simulink model "NL_Corner_FIw"  (R2016b)
settings: Solver=FixedStepAuto  StartTime=0.0  StopTime=5  FixedStep=0.001  RelTol=1e-3
values from neighbouring files (symbols this model uses):
  AccelError = eye(3)    [SimulinkInit.m]
  C_psi = 3.1176e-5    (= 3.1176e-05)    [ParameterInit.m]
  control_system = CS_LQR    (= 1)    [SimulinkInit.m]
  dPhiMat = [cos(phi_30)/cos(phi_20), -sin(phi_30)/cos(phi_20), 0 ... (first row only)    [ParameterInit.m]
  g = 9.81    [ParameterInit.m]
  GyroError = eye(3)    [SimulinkInit.m]
  I_K_inv = inv(I_K)    [ParameterInit.m]
  I_KO = I_GHO + m_R*(eye(3)*dot(r_1,r_1)-r_1*r_1')                 + m_R*(eye(3)*dot(r_2,r_2)-r_2*r_2')                 + m_R*(eye(3)*dot(r_3,r_3)-r_3*r_3')    [ParameterInit.m]
  I_R1M1 = [3.358e-4, 0, 0; 0, 1.961e-4, 0; 0, 0, 1.681e-4]    [ParameterInit.m]
  I_R2M2 = [1.691e-4, 0, 0; 0, 3.358e-4, 0; 0, 0, 1.961e-4]    [ParameterInit.m]
  I_R3M3 = [1.961e-4, 0, 0; 0, 1.691e-4, 0; 0, 0, 3.358e-4]    [ParameterInit.m]
  I_R_inv = inv(I_R)    [ParameterInit.m]
  Kd = K_unlimited    [LinearSimulationScript.m]    (also in controller_design_lqr.m = KKd * [eye(7), zeros(7,2)]/T_K)
  l_C = 0.066    [ParameterInit.m]
  m = 1.532    [ParameterInit.m]
  phi0 = x0(1:3) + [0; phi_20; phi_30]    [SimulinkInit.m]
  phi_20 = -2*atan(sqrt(2)-sqrt(3))    [ParameterInit.m]
  phi_30 = -pi/4    (= -0.785398163397)    [ParameterInit.m]
  saturation_select = SATURATION_OFF    [LinearSimulationScript.m]    (also in SimulinkInit.m = 2)
  Ta = 0.02    [ParameterInit.m]
  u_K0 = x0(4:6)    [SimulinkInit.m]
  u_R0 = x0(7:9)    [SimulinkInit.m]
  x0 = [0; 0.11; 0.08; 0; 1; -2; 3; -16; 0]    [LinearSimulationScript.m]    (also in SimulinkInit.m = [0; 0.05; 0.02; 0; 0; 0; 0; 0; 0])
  x_offset = [0; 0.02; 0.0; 0; 0; 0; 0; 0; 0]    [SimulinkInit.m]
libraries: vrlib x4, simulink x1
settings Model: Creator=michael  LastModifiedBy=ich

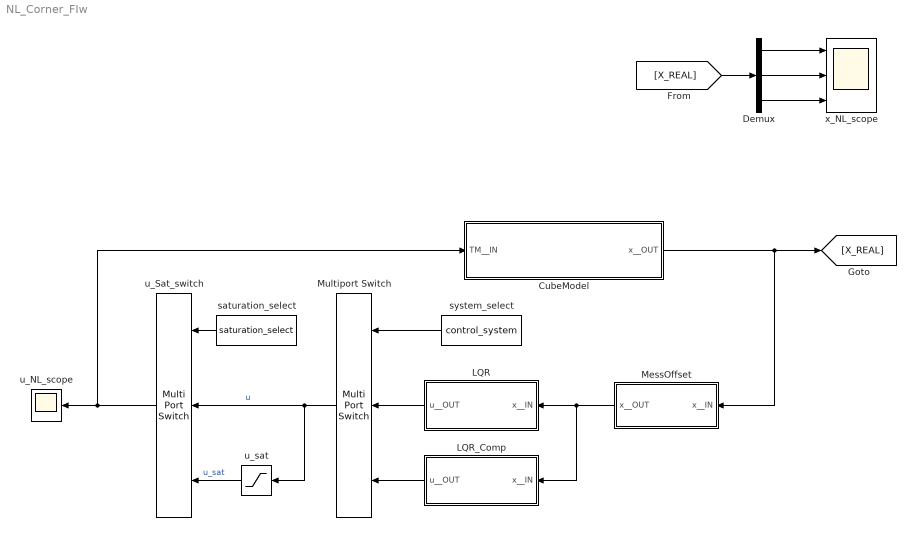
== system NL_Corner_FIw ==
  CubeModel : Subsystem
  Demux : Demux  Outputs=3
  LQR : Subsystem
  LQR_Comp : Subsystem
  MessOffset : Subsystem
  Multiport Switch : MultiPortSwitch  Inputs=2
  saturation_select : Constant  Value=saturation_select
  system_select : Constant  Value=control_system
  u_NL_scope : Scope
  u_Sat_switch : MultiPortSwitch  Inputs=2
  u_sat : Saturate  UpperLimit=0.1  LowerLimit=-0.1
  x_NL_scope : Scope  NumInputPorts=3
  wires:
  MessOffset/1(x__OUT) -> LQR/1(x__IN), LQR_Comp/1(x__IN)
  CubeModel/1(x__OUT) -> [X_REAL], MessOffset/1(x__IN)
  [X_REAL] -> Demux/1
  Demux/1 -> x_NL_scope/1
  Demux/2 -> x_NL_scope/2
  Demux/3 -> x_NL_scope/3
  LQR/1(u__OUT) -> Multiport Switch/2
  LQR_Comp/1(u__OUT) -> Multiport Switch/3
  system_select/1 -> Multiport Switch/1
  u_sat/1 -> u_Sat_switch/3  "u_sat"
  Multiport Switch/1 -> u_Sat_switch/2, u_sat/1  "u"
  saturation_select/1 -> u_Sat_switch/1
  u_Sat_switch/1 -> CubeModel/1(TM__IN), u_NL_scope/1

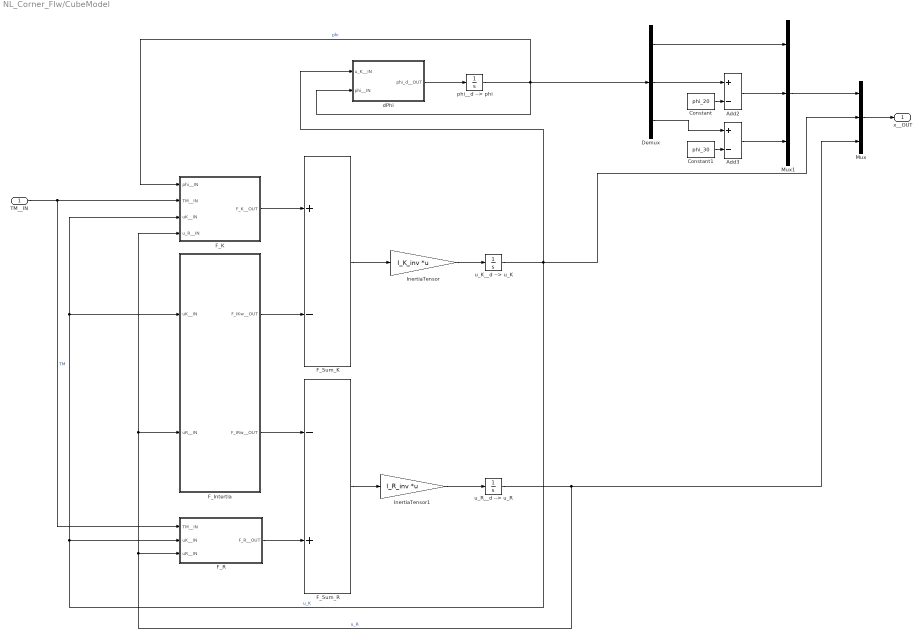
== system NL_Corner_FIw/CubeModel ==
  TM__IN : Inport
  Add2 : Sum  Inputs=+-
  Add3 : Sum  Inputs=+-
  Constant : Constant  Value=phi_20
  Constant1 : Constant  Value=phi_30
  Demux : Demux  Outputs=3
  F_Intertia : Subsystem
  F_K : Subsystem
  F_R : Subsystem
  F_Sum_K : Sum  Inputs=+-
  F_Sum_R : Sum  Inputs=-+
  InertiaTensor : Gain  Gain=I_K_inv  Multiplication=Matrix(K*u) (u vector)
  InertiaTensor1 : Gain  Gain=I_R_inv  Multiplication=Matrix(K*u) (u vector)
  Mux : Mux  Inputs=3
  Mux1 : Mux  Inputs=3
  dPhi : Subsystem
  phi__d --> phi : Integrator  InitialCondition=phi0
  u_K__d --> u_K : Integrator  InitialCondition=u_K0
  u_R__d --> u_R : Integrator  InitialCondition=u_R0
  x__OUT : Outport
  wires:
  u_K__d --> u_K/1 -> F_R/2(uK__IN), F_Intertia/1(uK__IN), F_K/3(uK__IN), dPhi/1(u_K__IN), Mux/2  "u_K"
  u_R__d --> u_R/1 -> F_R/3(uR__IN), F_Intertia/2(uR__IN), F_K/4(u_R__IN), Mux/3  "u_R"
  dPhi/1(phi_d__OUT) -> phi__d --> phi/1
  Mux/1 -> x__OUT/1
  phi__d --> phi/1 -> dPhi/2(phi__IN), F_K/1(phi__IN), Demux/1  "phi"
  Demux/2 -> Add2/1
  Demux/3 -> Add3/1
  Constant1/1 -> Add3/2
  Constant/1 -> Add2/2
  Demux/1 -> Mux1/1
  Add2/1 -> Mux1/2
  Add3/1 -> Mux1/3
  Mux1/1 -> Mux/1
  F_K/1(F_K__OUT) -> F_Sum_K/1
  F_Sum_K/1 -> InertiaTensor/1
  F_R/1(F_R__OUT) -> F_Sum_R/2
  F_Sum_R/1 -> InertiaTensor1/1
  InertiaTensor/1 -> u_K__d --> u_K/1
  InertiaTensor1/1 -> u_R__d --> u_R/1
  TM__IN/1 -> F_K/2(TM__IN), F_R/1(TM__IN)  "TM"
  F_Intertia/2(F_IRw__OUT) -> F_Sum_R/1
  F_Intertia/1(F_IKw__OUT) -> F_Sum_K/2

== system NL_Corner_FIw/LQR ==
  x__IN : Inport  SampleTime=Ta
  Gain : Gain  Gain=-Kd  Multiplication=Matrix(K*u) (u vector)
  u__OUT : Outport
  wires:
  x__IN/1 -> Gain/1
  Gain/1 -> u__OUT/1

== system NL_Corner_FIw/LQR_Comp ==
  x__IN : Inport  SampleTime=Ta
  CompFilter : Subsystem
  Gain : Gain  Gain=-Kd  Multiplication=Matrix(K*u) (u vector)
  u__OUT : Outport
  wires:
  x__IN/1 -> CompFilter/1(x__IN)
  Gain/1 -> u__OUT/1
  CompFilter/1(x__OUT) -> Gain/1

== system NL_Corner_FIw/MessOffset ==
  x__IN : Inport
  Add : Sum  Inputs=+++
  Band-Limited White Noise : simulink/Sources/Band-Limited White Noise  Cov=x_noise  Ts=0.1  seed=[1;2;3;4;5;6;7;8;9]
  Constant : Constant  Value=x_offset
  SensorTilt : Subsystem
  x__OUT : Outport
  wires:
  x__IN/1 -> SensorTilt/1(x__IN)
  Add/1 -> x__OUT/1
  Constant/1 -> Add/2
  Band-Limited White Noise/1 -> Add/3
  SensorTilt/1(x__OUT) -> Add/1

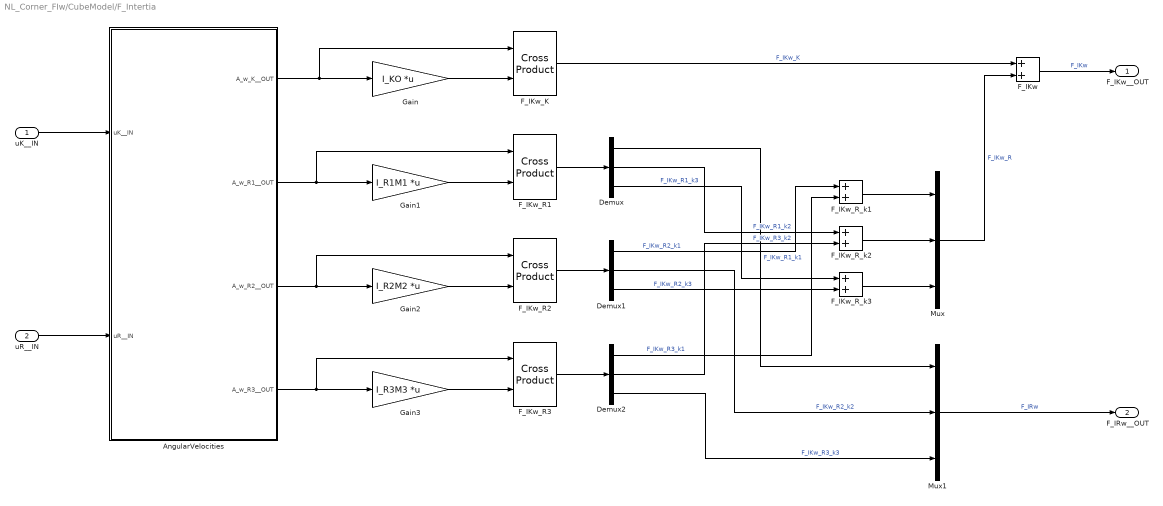
== system NL_Corner_FIw/CubeModel/F_Intertia ==
  uK__IN : Inport
  uR__IN : Inport  Port=2
  AngularVelocities : Subsystem
  Demux : Demux  Outputs=3
  Demux1 : Demux  Outputs=3
  Demux2 : Demux  Outputs=3
  F_IKw : Sum
  F_IKw_K : vrlib/Utilities/Cross Product
  F_IKw_R1 : vrlib/Utilities/Cross Product
  F_IKw_R2 : vrlib/Utilities/Cross Product
  F_IKw_R3 : vrlib/Utilities/Cross Product
  F_IKw_R_k1 : Sum
  F_IKw_R_k2 : Sum
  F_IKw_R_k3 : Sum
  Gain : Gain  Gain=I_KO  Multiplication=Matrix(K*u) (u vector)
  Gain1 : Gain  Gain=I_R1M1  Multiplication=Matrix(K*u) (u vector)
  Gain2 : Gain  Gain=I_R2M2  Multiplication=Matrix(K*u) (u vector)
  Gain3 : Gain  Gain=I_R3M3  Multiplication=Matrix(K*u) (u vector)
  Mux : Mux  Inputs=3
  Mux1 : Mux  Inputs=3
  F_IKw__OUT : Outport
  F_IRw__OUT : Outport  Port=2
  wires:
  uK__IN/1 -> AngularVelocities/1(uK__IN)
  uR__IN/1 -> AngularVelocities/2(uR__IN)
  AngularVelocities/1(A_w_K__OUT) -> F_IKw_K/1, Gain/1
  Gain/1 -> F_IKw_K/2
  AngularVelocities/2(A_w_R1__OUT) -> F_IKw_R1/1, Gain1/1
  Gain1/1 -> F_IKw_R1/2
  AngularVelocities/3(A_w_R2__OUT) -> Gain2/1, F_IKw_R2/1
  Gain2/1 -> F_IKw_R2/2
  AngularVelocities/4(A_w_R3__OUT) -> F_IKw_R3/1, Gain3/1
  Gain3/1 -> F_IKw_R3/2
  F_IKw_R1/1 -> Demux/1
  Demux/1 -> Mux1/1  "F_IKw_R1_k1"
  Demux/2 -> F_IKw_R_k2/1  "F_IKw_R1_k2"
  Demux/3 -> F_IKw_R_k3/1  "F_IKw_R1_k3"
  F_IKw_R2/1 -> Demux1/1
  Demux1/1 -> F_IKw_R_k1/1  "F_IKw_R2_k1"
  Demux1/2 -> Mux1/2  "F_IKw_R2_k2"
  Demux1/3 -> F_IKw_R_k3/2  "F_IKw_R2_k3"
  F_IKw_R3/1 -> Demux2/1
  Demux2/1 -> F_IKw_R_k1/2  "F_IKw_R3_k1"
  Demux2/2 -> F_IKw_R_k2/2  "F_IKw_R3_k2"
  Demux2/3 -> Mux1/3  "F_IKw_R3_k3"
  F_IKw_R_k1/1 -> Mux/1
  F_IKw_R_k3/1 -> Mux/3
  F_IKw_R_k2/1 -> Mux/2
  Mux/1 -> F_IKw/2  "F_IKw_R"
  F_IKw_K/1 -> F_IKw/1  "F_IKw_K"
  F_IKw/1 -> F_IKw__OUT/1  "F_IKw"
  Mux1/1 -> F_IRw__OUT/1  "F_IRw"

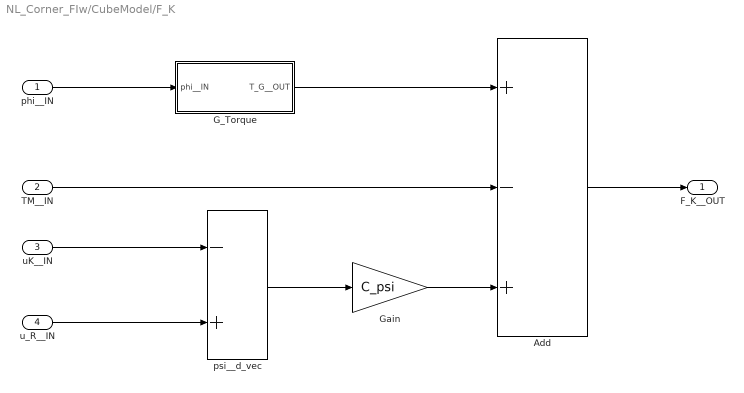
== system NL_Corner_FIw/CubeModel/F_K ==
  phi__IN : Inport
  TM__IN : Inport  Port=2
  uK__IN : Inport  Port=3
  u_R__IN : Inport  Port=4
  Add : Sum  Inputs=+-+
  G_Torque : Subsystem
  Gain : Gain  Gain=C_psi
  psi__d_vec : Sum  Inputs=-+
  F_K__OUT : Outport
  wires:
  phi__IN/1 -> G_Torque/1(phi__IN)
  uK__IN/1 -> psi__d_vec/1
  u_R__IN/1 -> psi__d_vec/2
  psi__d_vec/1 -> Gain/1
  G_Torque/1(T_G__OUT) -> Add/1
  Gain/1 -> Add/3
  TM__IN/1 -> Add/2
  Add/1 -> F_K__OUT/1

== system NL_Corner_FIw/CubeModel/F_R ==
  TM__IN : Inport
  uK__IN : Inport  Port=2
  uR__IN : Inport  Port=3
  Gain : Gain  Gain=C_psi
  TorqueSum : Sum  Inputs=+-
  psi__d_vec : Sum  Inputs=-+
  F_R__OUT : Outport
  wires:
  uR__IN/1 -> psi__d_vec/2
  uK__IN/1 -> psi__d_vec/1
  psi__d_vec/1 -> Gain/1
  TM__IN/1 -> TorqueSum/1
  Gain/1 -> TorqueSum/2
  TorqueSum/1 -> F_R__OUT/1  "F_R"

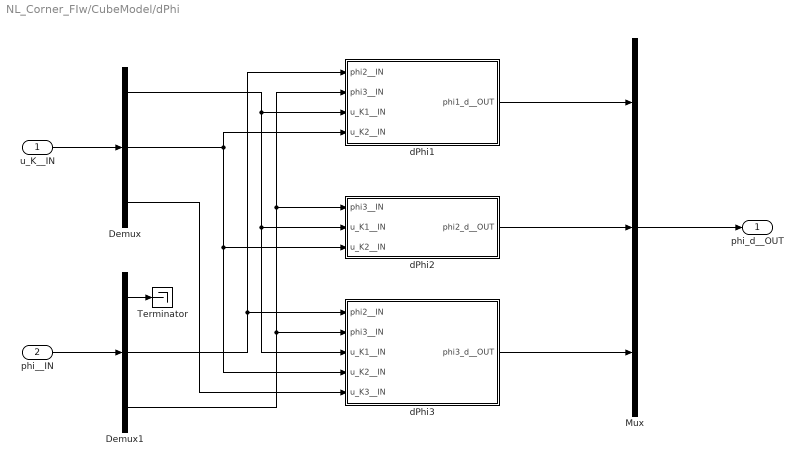
== system NL_Corner_FIw/CubeModel/dPhi ==
  u_K__IN : Inport
  phi__IN : Inport  Port=2
  Demux : Demux  Outputs=3
  Demux1 : Demux  Outputs=3
  Mux : Mux  Inputs=3
  Terminator : Terminator
  dPhi1 : Subsystem
  dPhi2 : Subsystem
  dPhi3 : Subsystem
  phi_d__OUT : Outport
  wires:
  u_K__IN/1 -> Demux/1
  Mux/1 -> phi_d__OUT/1
  phi__IN/1 -> Demux1/1
  dPhi1/1(phi1_d__OUT) -> Mux/1
  dPhi2/1(phi2_d__OUT) -> Mux/2
  dPhi3/1(phi3_d__OUT) -> Mux/3
  Demux1/2 -> dPhi3/1(phi2__IN), dPhi1/1(phi2__IN)
  Demux1/3 -> dPhi3/2(phi3__IN), dPhi2/1(phi3__IN), dPhi1/2(phi3__IN)
  Demux1/1 -> Terminator/1
  Demux/2 -> dPhi2/3(u_K2__IN), dPhi3/4(u_K2__IN), dPhi1/4(u_K2__IN)
  Demux/3 -> dPhi3/5(u_K3__IN)
  Demux/1 -> dPhi1/3(u_K1__IN), dPhi2/2(u_K1__IN), dPhi3/3(u_K1__IN)

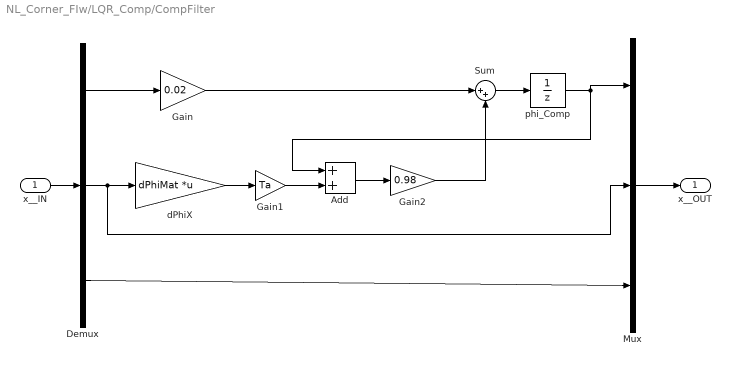
== system NL_Corner_FIw/LQR_Comp/CompFilter ==
  x__IN : Inport
  Add : Sum
  Demux : Demux  Outputs=3
  Gain : Gain  Gain=0.02
  Gain1 : Gain  Gain=Ta
  Gain2 : Gain  Gain=0.98
  Mux : Mux  Inputs=3
  Sum : Sum  Inputs=|++
  dPhiX : Gain  Gain=dPhiMat  Multiplication=Matrix(K*u) (u vector)
  phi_Comp : UnitDelay  InitialCondition=x0(1:3)  SampleTime=0.02
  x__OUT : Outport
  wires:
  x__IN/1 -> Demux/1
  Demux/1 -> Gain/1
  Demux/2 -> Mux/2, dPhiX/1
  dPhiX/1 -> Gain1/1
  Gain1/1 -> Add/2
  Add/1 -> Gain2/1
  Gain/1 -> Sum/1
  Gain2/1 -> Sum/2
  Sum/1 -> phi_Comp/1
  phi_Comp/1 -> Add/1, Mux/1
  Mux/1 -> x__OUT/1
  Demux/3 -> Mux/3

== system NL_Corner_FIw/MessOffset/SensorTilt ==
  x__IN : Inport
  Demux : Demux  Outputs=3
  Gain : Gain  Gain=GyroError  Multiplication=Matrix(K*u) (u vector)
  Gain1 : Gain  Gain=AccelError  Multiplication=Matrix(K*u) (u vector)
  Mux : Mux  Inputs=3
  x__OUT : Outport
  wires:
  x__IN/1 -> Demux/1
  Demux/2 -> Gain/1
  Mux/1 -> x__OUT/1
  Gain/1 -> Mux/2
  Demux/1 -> Gain1/1
  Demux/3 -> Mux/3
  Gain1/1 -> Mux/1

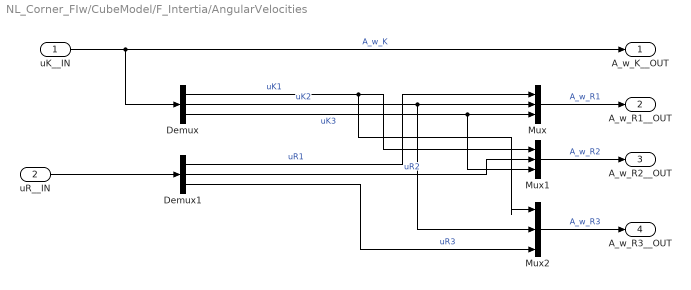
== system NL_Corner_FIw/CubeModel/F_Intertia/AngularVelocities ==
  uK__IN : Inport
  uR__IN : Inport  Port=2
  Demux : Demux  Outputs=3
  Demux1 : Demux  Outputs=3
  Mux : Mux  Inputs=3
  Mux1 : Mux  Inputs=3
  Mux2 : Mux  Inputs=3
  A_w_K__OUT : Outport
  A_w_R1__OUT : Outport  Port=2
  A_w_R2__OUT : Outport  Port=3
  A_w_R3__OUT : Outport  Port=4
  wires:
  uK__IN/1 -> Demux/1, A_w_K__OUT/1  "A_w_K"
  Mux/1 -> A_w_R1__OUT/1  "A_w_R1"
  Mux1/1 -> A_w_R2__OUT/1  "A_w_R2"
  Mux2/1 -> A_w_R3__OUT/1  "A_w_R3"
  Demux/2 -> Mux2/2, Mux/2  "uK2"
  Demux/3 -> Mux1/3, Mux/3  "uK3"
  Demux/1 -> Mux2/1, Mux1/1  "uK1"
  uR__IN/1 -> Demux1/1
  Demux1/1 -> Mux/1  "uR1"
  Demux1/2 -> Mux1/2  "uR2"
  Demux1/3 -> Mux2/3  "uR3"

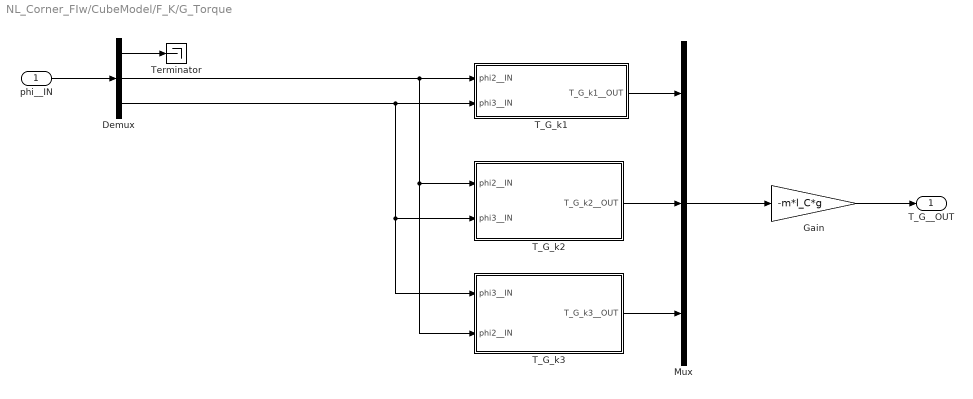
== system NL_Corner_FIw/CubeModel/F_K/G_Torque ==
  phi__IN : Inport
  Demux : Demux  Outputs=3
  Gain : Gain  Gain=-m*l_C*g
  Mux : Mux  Inputs=3
  T_G_k1 : Subsystem
  T_G_k2 : Subsystem
  T_G_k3 : Subsystem
  Terminator : Terminator
  T_G__OUT : Outport
  wires:
  phi__IN/1 -> Demux/1
  Demux/1 -> Terminator/1
  Demux/2 -> T_G_k3/2(phi2__IN), T_G_k2/1(phi2__IN), T_G_k1/1(phi2__IN)
  Demux/3 -> T_G_k3/1(phi3__IN), T_G_k2/2(phi3__IN), T_G_k1/2(phi3__IN)
  T_G_k3/1(T_G_k3__OUT) -> Mux/3
  Mux/1 -> Gain/1
  T_G_k2/1(T_G_k2__OUT) -> Mux/2
  T_G_k1/1(T_G_k1__OUT) -> Mux/1
  Gain/1 -> T_G__OUT/1

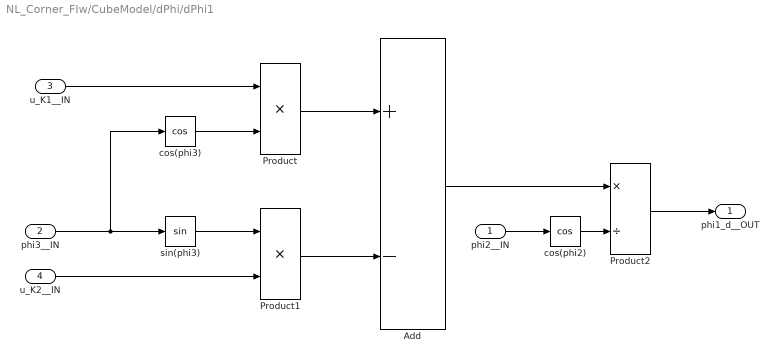
== system NL_Corner_FIw/CubeModel/dPhi/dPhi1 ==
  phi2__IN : Inport
  phi3__IN : Inport  Port=2
  u_K1__IN : Inport  Port=3
  u_K2__IN : Inport  Port=4
  Add : Sum  Inputs=+-
  Product : Product  Inputs=**
  Product1 : Product  Inputs=**
  Product2 : Product  Inputs=*/
  cos(phi2) : Trigonometry  Operator=cos
  cos(phi3) : Trigonometry  Operator=cos
  sin(phi3) : Trigonometry
  phi1_d__OUT : Outport
  wires:
  phi3__IN/1 -> cos(phi3)/1, sin(phi3)/1
  cos(phi3)/1 -> Product/2
  u_K1__IN/1 -> Product/1
  sin(phi3)/1 -> Product1/1
  u_K2__IN/1 -> Product1/2
  Product/1 -> Add/1
  Product1/1 -> Add/2
  phi2__IN/1 -> cos(phi2)/1
  Add/1 -> Product2/1
  cos(phi2)/1 -> Product2/2
  Product2/1 -> phi1_d__OUT/1

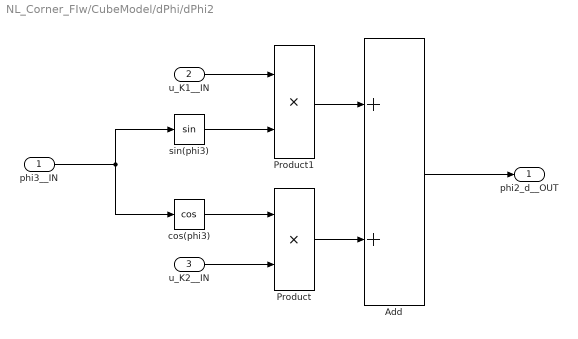
== system NL_Corner_FIw/CubeModel/dPhi/dPhi2 ==
  phi3__IN : Inport
  u_K1__IN : Inport  Port=2
  u_K2__IN : Inport  Port=3
  Add : Sum
  Product : Product
  Product1 : Product
  cos(phi3) : Trigonometry  Operator=cos
  sin(phi3) : Trigonometry
  phi2_d__OUT : Outport
  wires:
  phi3__IN/1 -> sin(phi3)/1, cos(phi3)/1
  cos(phi3)/1 -> Product/1
  u_K2__IN/1 -> Product/2
  u_K1__IN/1 -> Product1/1
  sin(phi3)/1 -> Product1/2
  Product1/1 -> Add/1
  Product/1 -> Add/2
  Add/1 -> phi2_d__OUT/1

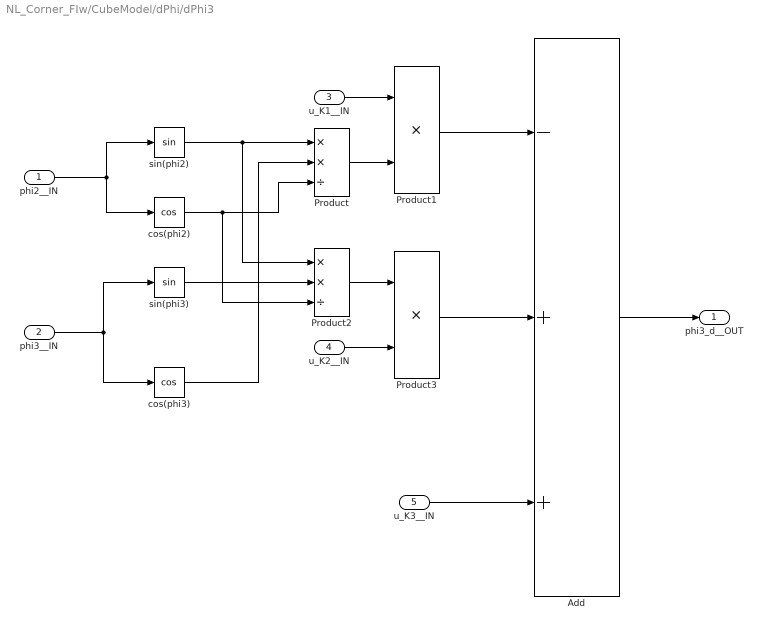
== system NL_Corner_FIw/CubeModel/dPhi/dPhi3 ==
  phi2__IN : Inport
  phi3__IN : Inport  Port=2
  u_K1__IN : Inport  Port=3
  u_K2__IN : Inport  Port=4
  u_K3__IN : Inport  Port=5
  Add : Sum  Inputs=-++
  Product : Product  Inputs=**/
  Product1 : Product
  Product2 : Product  Inputs=**/
  Product3 : Product
  cos(phi2) : Trigonometry  Operator=cos
  cos(phi3) : Trigonometry  Operator=cos
  sin(phi2) : Trigonometry
  sin(phi3) : Trigonometry
  phi3_d__OUT : Outport
  wires:
  phi2__IN/1 -> cos(phi2)/1, sin(phi2)/1
  phi3__IN/1 -> cos(phi3)/1, sin(phi3)/1
  sin(phi2)/1 -> Product2/1, Product/1
  cos(phi3)/1 -> Product/2
  u_K1__IN/1 -> Product1/1
  Product/1 -> Product1/2
  cos(phi2)/1 -> Product2/3, Product/3
  sin(phi3)/1 -> Product2/2
  Product2/1 -> Product3/1
  u_K2__IN/1 -> Product3/2
  Product1/1 -> Add/1
  Product3/1 -> Add/2
  u_K3__IN/1 -> Add/3
  Add/1 -> phi3_d__OUT/1

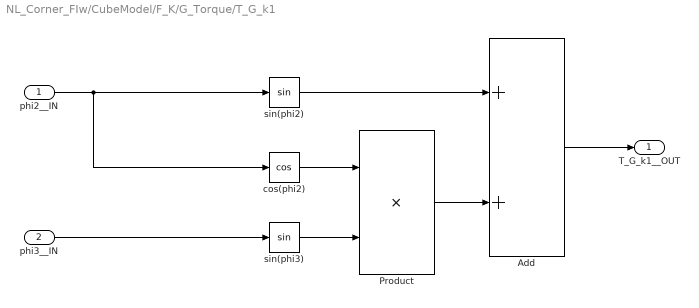
== system NL_Corner_FIw/CubeModel/F_K/G_Torque/T_G_k1 ==
  phi2__IN : Inport
  phi3__IN : Inport  Port=2
  Add : Sum
  Product : Product
  cos(phi2) : Trigonometry  Operator=cos
  sin(phi2) : Trigonometry
  sin(phi3) : Trigonometry
  T_G_k1__OUT : Outport
  wires:
  phi2__IN/1 -> cos(phi2)/1, sin(phi2)/1
  cos(phi2)/1 -> Product/1
  sin(phi2)/1 -> Add/1
  Product/1 -> Add/2
  phi3__IN/1 -> sin(phi3)/1
  sin(phi3)/1 -> Product/2
  Add/1 -> T_G_k1__OUT/1

== system NL_Corner_FIw/CubeModel/F_K/G_Torque/T_G_k2 ==
  phi2__IN : Inport
  phi3__IN : Inport  Port=2
  Add : Sum  Inputs=-+
  Product : Product
  cos(phi2) : Trigonometry  Operator=cos
  cos(phi3) : Trigonometry  Operator=cos
  sin(phi2) : Trigonometry
  T_G_k2__OUT : Outport
  wires:
  sin(phi2)/1 -> Add/1
  phi2__IN/1 -> cos(phi2)/1, sin(phi2)/1
  cos(phi2)/1 -> Product/1
  Add/1 -> T_G_k2__OUT/1
  phi3__IN/1 -> cos(phi3)/1
  cos(phi3)/1 -> Product/2
  Product/1 -> Add/2

== system NL_Corner_FIw/CubeModel/F_K/G_Torque/T_G_k3 ==
  phi3__IN : Inport
  phi2__IN : Inport  Port=2
  Add : Sum  Inputs=--
  Product : Product
  cos(phi2) : Trigonometry  Operator=cos
  cos(phi3) : Trigonometry  Operator=cos
  sin(phi3) : Trigonometry
  T_G_k3__OUT : Outport
  wires:
  Product/1 -> T_G_k3__OUT/1
  phi3__IN/1 -> cos(phi3)/1, sin(phi3)/1
  phi2__IN/1 -> cos(phi2)/1
  cos(phi3)/1 -> Add/2
  cos(phi2)/1 -> Product/2
  sin(phi3)/1 -> Add/1
  Add/1 -> Product/1
